simulink model "AFPSM"  (R2018a)
settings: Solver=ode15s  StartTime=0.0  StopTime=5.0  RelTol=1e-3
InitFcn:
  | Pref=2000;
  | D=4;
  | P=10;
  | Rd=5;
  | Rq=5;
  | Ld=2.094;
  | Lq= 0.8187;
  | Phi= 1.6
  | Pref = 2000;
  | J=4;
  | K=0.16;
  | c1= 0.5176;
  | c2= 116;
  | c3= 0.4;
  | c4= 5;
  | c5= 21;
  | c6= 0.0068;
  | Den= 1.225;
  | A= 2
libraries: powerlib x29, simulink x6, powerlib_meascontrol x3
settings Model: Creator=samue  LastModifiedBy=samue

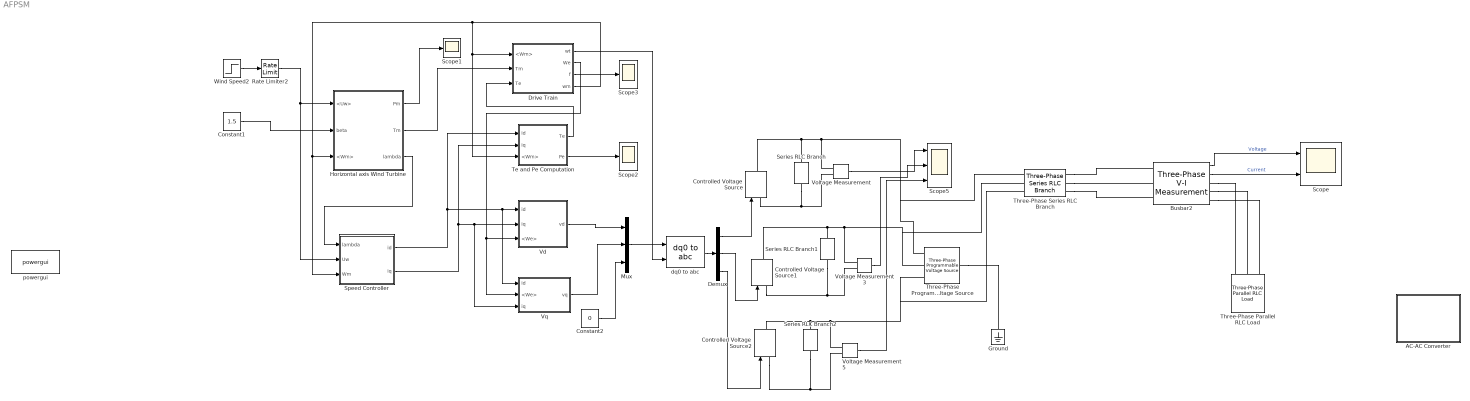
== system AFPSM ==
  AC-AC Converter : Subsystem
  Busbar2 : powerlib/Measurements/Three-Phase V-I Measurement  VoltageMeasurement=phase-to-phase  SetLabelV=off  LabelV=Vabc  Vpu=off  VpuLL=off  CurrentMeasurement=yes  SetLabelI=off  LabelI=Iabc  Ipu=off  Pbase=100e6  Vbase=500e3  OutputType=Complex  PhasorSimulation=off  PSBequivalent=0
  Constant1 : Constant  Value=1.5
  Constant2 : Constant  Value=0
  Controlled Voltage Source : powerlib/Electrical Sources/Controlled Voltage Source  Initialize=on  Source_Type=AC  Amplitude=0  Phase=0  Frequency=60  Measurements=None
  Controlled Voltage Source1 : powerlib/Electrical Sources/Controlled Voltage Source  Initialize=on  Source_Type=AC  Amplitude=0  Phase=0  Frequency=60  Measurements=None
  Controlled Voltage Source2 : powerlib/Electrical Sources/Controlled Voltage Source  Initialize=on  Source_Type=AC  Amplitude=0  Phase=0  Frequency=60  Measurements=None
  Demux : Demux  Outputs=3
  Drive Train : Subsystem
  Ground : powerlib/Elements/Ground  LConnTagsString=a
  Horizontal axis Wind Turbine : Subsystem
  Mux : Mux  Inputs=3
  Rate Limiter2 : RateLimiter
  Scope : Scope  NumInputPorts=2
  Scope1 : Scope
  Scope2 : Scope
  Scope3 : Scope
  Scope5 : Scope  NumInputPorts=3
  Series RLC Branch : powerlib/Elements/Series RLC Branch  LConnTagsString=__new0  RConnTagsString=__new0  BranchType=R  Resistance=1  Inductance=1e-3  SetiL0=off  InitialCurrent=0  Capacitance=1e-6  Setx0=off  InitialVoltage=0  Measurements=None
  Series RLC Branch1 : powerlib/Elements/Series RLC Branch  LConnTagsString=__new0  RConnTagsString=__new0  BranchType=R  Resistance=1  Inductance=1e-3  SetiL0=off  InitialCurrent=0  Capacitance=1e-6  Setx0=off  InitialVoltage=0  Measurements=None
  Series RLC Branch2 : powerlib/Elements/Series RLC Branch  LConnTagsString=__new0  RConnTagsString=__new0  BranchType=R  Resistance=1  Inductance=1e-3  SetiL0=off  InitialCurrent=0  Capacitance=1e-6  Setx0=off  InitialVoltage=0  Measurements=None
  Speed Controller : Subsystem
  Te and Pe Computation : Subsystem
  Three-Phase Parallel RLC Load : powerlib/Elements/Three-Phase Parallel RLC Load  LConnTagsString=A|B|C  Configuration=Y (grounded)  NominalVoltage=1000  Vabc=[1e3 1e3 1e3]  Vabcp=[1e3 1e3 1e3]  NominalFrequency=60  UnbalancedPower=off  ActivePower=10e3  InductivePower=0  CapacitivePower=0  Pabc=[10e3 9e3 11e3]  QLabc=[100 90 110]  QCabc=[100 90 110]  Pabcp=[10e3 9e3 11e3]  QLabcp=[100 90 110]  QCabcp=[100 90 110]  Measurements=None  LoadType=constant Z
  Three-Phase Programmable Voltage Source : powerlib/Electrical Sources/Three-Phase Programmable Voltage Source  PositiveSequence="[100  0 60]"  VariationEntity=None  VariationType=Table of time-amplitude pairs  VariationTypeAlt=Step  VariationStep=0.5  VariationRate=10  VariationMagnitude=0.3  VariationFrequency=2  VariationTiming=[1 2]  VariationPhaseA=off  Amplitudes=[1 0.8 1.2 1.0]  TimeValues=[0 0.1 0.15 0.2]  HarmonicGeneration=off  HarmonicA=[3 0.2 -25 0]  HarmonicB=[2 0.15 35 2]  Timing="[0.05  3]"  BusType=swing  Pref=0  Qref=0  Qmin=-inf  Qmax=inf
  Three-Phase Series RLC Branch : powerlib/Elements/Three-Phase Series RLC Branch  LConnTagsString=A|B|C  RConnTagsString=A|B|C  BranchType=RL  Resistance=1  Inductance=1e-3  Capacitance=1e-6  Measurements=None
  Vd : Subsystem
  Voltage Measurement : powerlib/Measurements/Voltage Measurement  PhasorSimulation=off  OutputType=Complex  PSBequivalent=0
  Voltage Measurement3 : powerlib/Measurements/Voltage Measurement  PhasorSimulation=off  OutputType=Complex  PSBequivalent=0
  Voltage Measurement5 : powerlib/Measurements/Voltage Measurement  PhasorSimulation=off  OutputType=Complex  PSBequivalent=0
  Vq : Subsystem
  Wind Speed2 : Step  Time=2  Before=6  After=15  SampleTime=0
  dq0 to abc : powerlib_meascontrol/Transformations/dq0 to abc  Alignment=90 degrees behind phase A axis
  powergui : powerlib/powergui  Priority=1  SimulationMode=Discrete  SampleTime=50e-6  frequency=60  Iterations=50  frequencyindice=60  Pbase=100e6  ErrMax=1e-4  UnitsV=kV  UnitsW=MW  buscounter=0  FunctionMessages=off  echomessages=off  EnableUseOfTLC=off  CurrentSourceSwitches=off  DisableSnubberDevices=off  DisableRonSwitches=off  DisableVfSwitches=off  DisplayEquations=off  SolverType=Tustin/Backward Euler (TBE)  Interpol=off  ExternalGateDelay=off  methode=off  Ts=100  x0status=blocks  SPID=on  SwTol=0  HookPort=off  RestoreLinks=warning  ResistiveCurrentMeasurement=off  Frange=[0:2:500]  Ylog=off  Xlog=on  ShowGrid=off  save=off  variable=ZData  structure=0  ZoomFFT=off  StartTime=0.0  cycles=1  DisplayStyle=1  fundamental=60  FreqAxis=off  MaxFrequency=1000  frequencyindicesteady=1  RmsSteady=1  display=off
  wires:
  Wind Speed2/1 -> Rate Limiter2/1
  Rate Limiter2/1 -> Speed Controller/2(Uw), Horizontal axis Wind Turbine/1(<Uw>)
  Horizontal axis Wind Turbine/3(lambda) -> Speed Controller/1(lambda)
  Horizontal axis Wind Turbine/2(Tm) -> Drive Train/2(Tm)
  Drive Train/2(We) -> Vd/3(<We>), Vq/2(<We>)
  Speed Controller/1(id) -> Vq/1(id), Vd/1(id), Te and Pe Computation/1(id)
  Speed Controller/2(iq) -> Vq/3(iq), Vd/2(iq), Te and Pe Computation/2(iq)
  Drive Train/4(wm) -> Speed Controller/3(Wm), Horizontal axis Wind Turbine/3(<Wm>), Drive Train/1(<Wm>), Te and Pe Computation/3(<Wm>)
  Te and Pe Computation/1(Te) -> Drive Train/3(Te)
  Constant1/1 -> Horizontal axis Wind Turbine/2(beta)
  Vd/1(vd) -> Mux/1
  Vq/1(vq) -> Mux/2
  Constant2/1 -> Mux/3
  Horizontal axis Wind Turbine/1(Pm) -> Scope1/1
  Drive Train/3(f) -> Scope3/1
  Mux/1 -> dq0 to abc/1
  Drive Train/1(wt) -> dq0 to abc/2
  Te and Pe Computation/2(Pe) -> Scope2/1
  dq0 to abc/1 -> Demux/1
  Demux/1 -> Controlled Voltage Source/1
  Demux/3 -> Controlled Voltage Source2/1
  Demux/2 -> Controlled Voltage Source1/1
  Voltage Measurement/1 -> Scope5/1
  Voltage Measurement3/1 -> Scope5/2
  Voltage Measurement5/1 -> Scope5/3
  Busbar2/2 -> Scope/2  "Current"
  Busbar2/1 -> Scope/1  "Voltage"
  connections:
  Three-Phase Programmable Voltage Source/LConn1 -- Ground/LConn1
  Voltage Measurement/LConn1 -- Three-Phase Series RLC Branch/LConn1 -- Three-Phase Programmable Voltage Source/RConn1 -- Controlled Voltage Source/RConn1 -- Series RLC Branch/LConn1
  Series RLC Branch/RConn1 -- Controlled Voltage Source/LConn1 -- Voltage Measurement/LConn2
  Voltage Measurement3/LConn1 -- Three-Phase Series RLC Branch/LConn2 -- Three-Phase Programmable Voltage Source/RConn2 -- Controlled Voltage Source1/RConn1 -- Series RLC Branch1/LConn1
  Controlled Voltage Source1/LConn1 -- Series RLC Branch1/RConn1 -- Voltage Measurement3/LConn2
  Voltage Measurement5/LConn1 -- Three-Phase Series RLC Branch/LConn3 -- Three-Phase Programmable Voltage Source/RConn3 -- Controlled Voltage Source2/RConn1 -- Series RLC Branch2/LConn1
  Controlled Voltage Source2/LConn1 -- Series RLC Branch2/RConn1 -- Voltage Measurement5/LConn2
  Busbar2/RConn3 -- Three-Phase Parallel RLC Load/LConn3
  Busbar2/RConn2 -- Three-Phase Parallel RLC Load/LConn2
  Busbar2/RConn1 -- Three-Phase Parallel RLC Load/LConn1
  Three-Phase Series RLC Branch/RConn1 -- Busbar2/LConn1
  Three-Phase Series RLC Branch/RConn2 -- Busbar2/LConn2
  Three-Phase Series RLC Branch/RConn3 -- Busbar2/LConn3

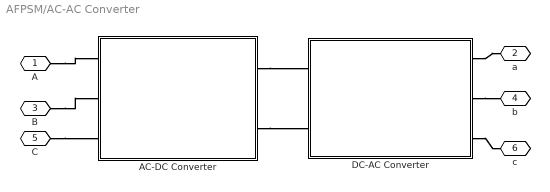
== system AFPSM/AC-AC Converter ==
  AC-DC Converter : Subsystem
  DC-AC Converter : Subsystem
  A : PMIOPort  Side=Left
  a : PMIOPort  Port=2  Side=Right
  B : PMIOPort  Port=3  Side=Left
  b : PMIOPort  Port=4  Side=Right
  C : PMIOPort  Port=5  Side=Left
  c : PMIOPort  Port=6  Side=Right
  connections:
  DC-AC Converter/RConn3 -- c/RConn1
  DC-AC Converter/RConn2 -- b/RConn1
  DC-AC Converter/RConn1 -- a/RConn1
  A/RConn1 -- AC-DC Converter/LConn1
  B/RConn1 -- AC-DC Converter/LConn2
  C/RConn1 -- AC-DC Converter/LConn3
  AC-DC Converter/RConn1 -- DC-AC Converter/LConn1
  AC-DC Converter/RConn2 -- DC-AC Converter/LConn2

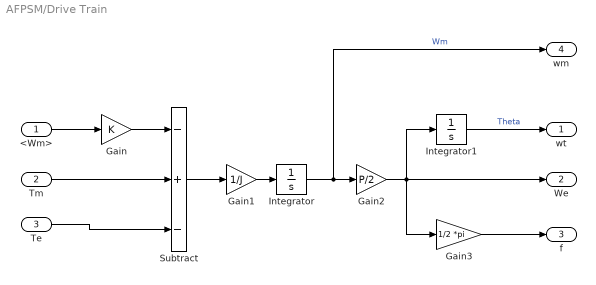
== system AFPSM/Drive Train ==
  <Wm> : Inport
  Tm : Inport  Port=2
  Te : Inport  Port=3
  Gain : Gain  Gain=K
  Gain1 : Gain  Gain=1/J
  Gain2 : Gain  Gain=P/2
  Gain3 : Gain  Gain=1/2 *pi
  Integrator : Integrator
  Integrator1 : Integrator
  Subtract : Sum  Inputs=-+-
  wt : Outport
  We : Outport  Port=2
  f : Outport  Port=3
  wm : Outport  Port=4
  wires:
  Tm/1 -> Subtract/2
  Integrator/1 -> wm/1, Gain2/1  "Wm"
  Gain/1 -> Subtract/1
  Gain2/1 -> We/1, Integrator1/1, Gain3/1
  Te/1 -> Subtract/3
  <Wm>/1 -> Gain/1
  Gain1/1 -> Integrator/1
  Subtract/1 -> Gain1/1
  Integrator1/1 -> wt/1  "Theta"
  Gain3/1 -> f/1

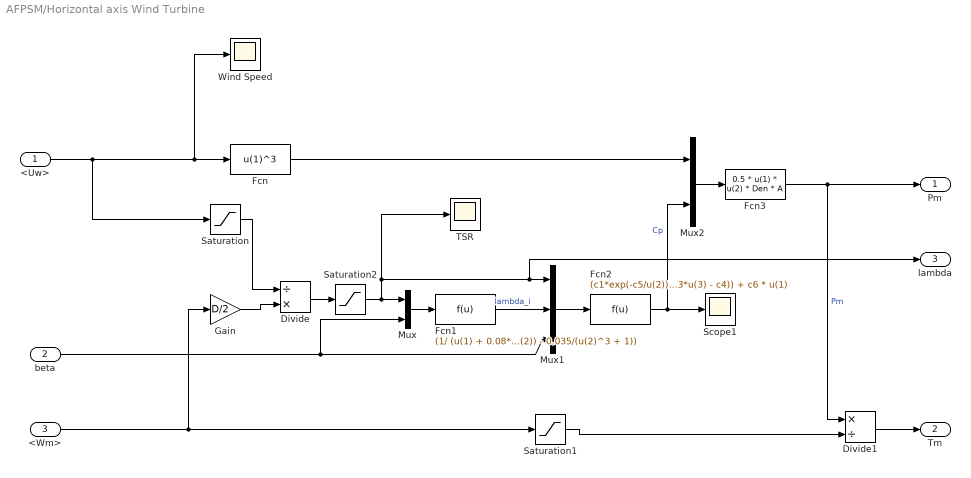
== system AFPSM/Horizontal axis Wind Turbine ==
  <Uw> : Inport
  beta : Inport  Port=2
  <Wm> : Inport  Port=3
  Divide : Product  Inputs=/*
  Divide1 : Product  Inputs=*/
  Fcn : Fcn  Expr=u(1)^3
  Fcn1 : Fcn  Expr=(1/ (u(1) + 0.08*u(2)) - 0.035/(u(2)^3 + 1))
  Fcn2 : Fcn  Expr=(c1*exp(-c5/u(2))*(c2/u(2) - c3*u(3) - c4)) + c6 * u(1)
  Fcn3 : Fcn  Expr=0.5 * u(1) * u(2) * Den * A
  Gain : Gain  Gain=D/2
  Mux : Mux  Inputs=2
  Mux1 : Mux  Inputs=3
  Mux2 : Mux  Inputs=2
  Saturation : Saturate
  Saturation1 : Saturate  UpperLimit=1e6  LowerLimit=1e-6
  Saturation2 : Saturate  UpperLimit=inf  LowerLimit=1e-6
  Scope1 : Scope
  TSR : Scope
  Wind Speed : Scope
  Pm : Outport
  Tm : Outport  Port=2
  lambda : Outport  Port=3
  wires:
  beta/1 -> Mux/2, Mux1/3
  Fcn2/1 -> Scope1/1, Mux2/2  "Cp"
  Divide/1 -> Saturation2/1
  Saturation2/1 -> Mux/1, lambda/1, Mux1/1, TSR/1
  Gain/1 -> Divide/2
  Fcn3/1 -> Pm/1, Divide1/1  "Pm"
  <Uw>/1 -> Saturation/1, Wind Speed/1, Fcn/1
  Mux/1 -> Fcn1/1
  Saturation1/1 -> Divide1/2
  Fcn1/1 -> Mux1/2  "lambda_i"
  <Wm>/1 -> Saturation1/1, Gain/1
  Mux1/1 -> Fcn2/1
  Mux2/1 -> Fcn3/1
  Fcn/1 -> Mux2/1
  Divide1/1 -> Tm/1
  Saturation/1 -> Divide/1

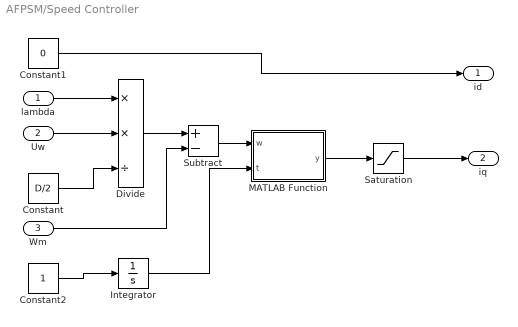
== system AFPSM/Speed Controller ==
  lambda : Inport
  Uw : Inport  Port=2
  Wm : Inport  Port=3
  Constant : Constant  Value=D/2
  Constant1 : Constant  Value=0
  Constant2 : Constant
  Divide : Product  Inputs=**/
  Integrator : Integrator
  MATLAB Function : MATLAB Function  TreatAsAtomicUnit=on
  Saturation : Saturate
  Subtract : Sum  Inputs=+-
  id : Outport
  iq : Outport  Port=2
  wires:
  MATLAB Function/1(y) -> Saturation/1
  Divide/1 -> Subtract/1
  Integrator/1 -> MATLAB Function/2(t)
  Saturation/1 -> iq/1
  Constant2/1 -> Integrator/1
  Constant/1 -> Divide/3
  Wm/1 -> Subtract/2
  Uw/1 -> Divide/2
  Constant1/1 -> id/1
  Subtract/1 -> MATLAB Function/1(w)
  lambda/1 -> Divide/1

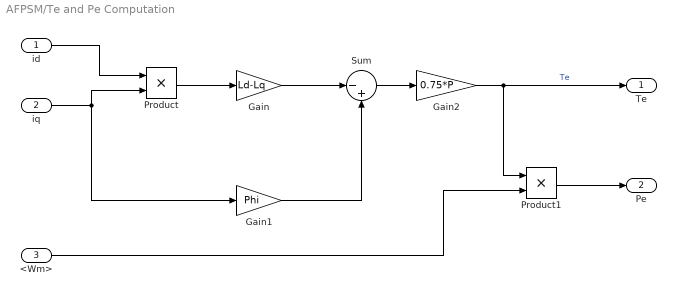
== system AFPSM/Te and Pe Computation ==
  id : Inport
  iq : Inport  Port=2
  <Wm> : Inport  Port=3
  Gain : Gain  Gain=Ld-Lq
  Gain1 : Gain  Gain=Phi
  Gain2 : Gain  Gain=0.75*P
  Product : Product
  Product1 : Product
  Sum : Sum  Inputs=|-+
  Te : Outport
  Pe : Outport  Port=2
  wires:
  <Wm>/1 -> Product1/2
  Product/1 -> Gain/1
  Sum/1 -> Gain2/1
  Gain/1 -> Sum/1
  Gain2/1 -> Te/1, Product1/1  "Te"
  Gain1/1 -> Sum/2
  Product1/1 -> Pe/1
  iq/1 -> Gain1/1, Product/2
  id/1 -> Product/1

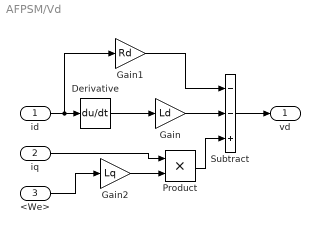
== system AFPSM/Vd ==
  id : Inport
  iq : Inport  Port=2
  <We> : Inport  Port=3
  Derivative : Derivative
  Gain : Gain  Gain=Ld
  Gain1 : Gain  Gain=Rd
  Gain2 : Gain  Gain=Lq
  Product : Product
  Subtract : Sum  Inputs=--+
  vd : Outport
  wires:
  Derivative/1 -> Gain/1
  Gain1/1 -> Subtract/1
  iq/1 -> Product/1
  Subtract/1 -> vd/1
  id/1 -> Gain1/1, Derivative/1
  Product/1 -> Subtract/3
  <We>/1 -> Gain2/1
  Gain/1 -> Subtract/2
  Gain2/1 -> Product/2

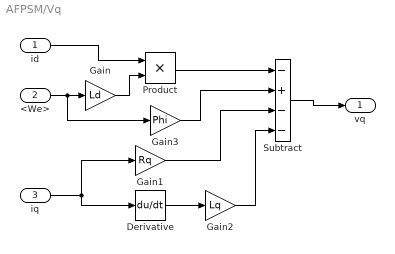
== system AFPSM/Vq ==
  id : Inport
  <We> : Inport  Port=2
  iq : Inport  Port=3
  Derivative : Derivative
  Gain : Gain  Gain=Ld
  Gain1 : Gain  Gain=Rq
  Gain2 : Gain  Gain=Lq
  Gain3 : Gain  Gain=Phi
  Product : Product
  Subtract : Sum  Inputs=-+--
  vq : Outport
  wires:
  iq/1 -> Gain1/1, Derivative/1
  Product/1 -> Subtract/1
  Gain/1 -> Product/2
  Subtract/1 -> vq/1
  <We>/1 -> Gain3/1, Gain/1
  id/1 -> Product/1
  Gain3/1 -> Subtract/2
  Gain1/1 -> Subtract/3
  Gain2/1 -> Subtract/4
  Derivative/1 -> Gain2/1

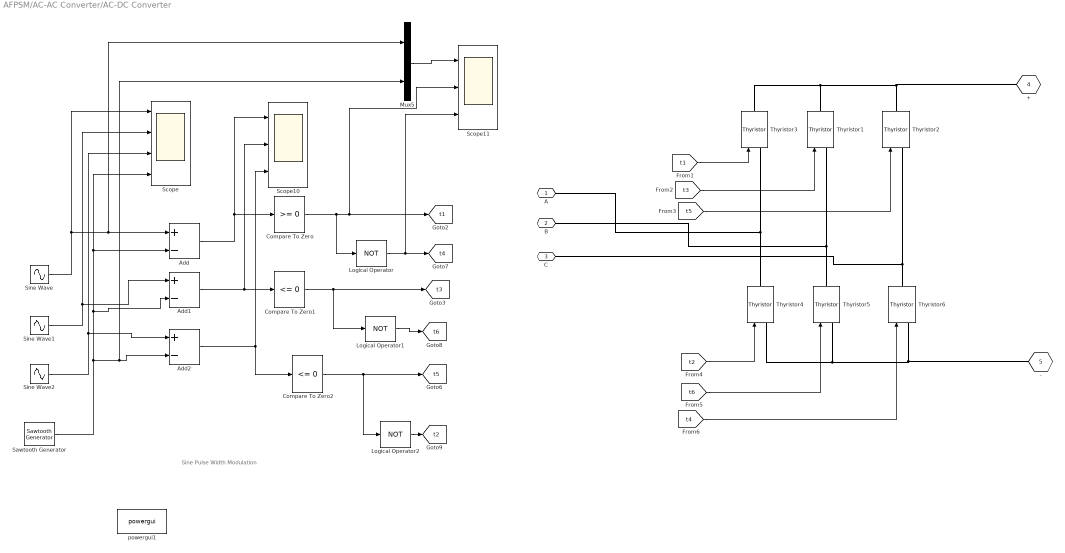
== system AFPSM/AC-AC Converter/AC-DC Converter ==
  note: Sine Pulse Width Modulation
  Add : Sum  Inputs=+-
  Add1 : Sum  Inputs=+-
  Add2 : Sum  Inputs=+-
  Compare To Zero : simulink/Logic and Bit Operations/Compare To Zero  relop=>=  OutDataTypeStr=boolean
  Compare To Zero1 : simulink/Logic and Bit Operations/Compare To Zero  relop=<=  OutDataTypeStr=boolean
  Compare To Zero2 : simulink/Logic and Bit Operations/Compare To Zero  relop=<=  OutDataTypeStr=boolean
  Logical Operator : Logic  Operator=NOT  AllPortsSameDT=off  OutDataTypeStr=boolean
  Logical Operator1 : Logic  Operator=NOT  AllPortsSameDT=off  OutDataTypeStr=boolean
  Logical Operator2 : Logic  Operator=NOT  AllPortsSameDT=off  OutDataTypeStr=boolean
  Mux5 : Mux  Inputs=2
  Sawtooth Generator : powerlib_meascontrol/Pulse & Signal Generators/Sawtooth Generator  Freq=10  Phase=180  Ts=0
      settings: SourceProductName=Simscape Power Systems
  Scope : Scope  NumInputPorts=4
  Scope10 : Scope  NumInputPorts=3
  Scope11 : Scope  NumInputPorts=3
  Sine Wave : Sin  Frequency=2*pi*60  SampleTime=0
  Sine Wave1 : Sin  Frequency=2*pi*60  Phase=(2*pi)/3  SampleTime=0
  Sine Wave2 : Sin  Frequency=2*pi*60  Phase=(-2*pi)/3  SampleTime=0
  Thyristor{1..6} (6 alike) : powerlib/Power Electronics/Thyristor  Ron=0.001  Lon=0  Vf=0.8  IC=0  Rs=500  Cs=250e-9  Measurements=off
  powergui1 : powerlib/powergui  Priority=1  SimulationMode=Continuous  SampleTime=50e-6  frequency=60  Iterations=50  frequencyindice=0  Pbase=100e6  ErrMax=1e-4  UnitsV=kV  UnitsW=MW  buscounter=0  FunctionMessages=off  echomessages=off  EnableUseOfTLC=off  CurrentSourceSwitches=off  DisableSnubberDevices=off  DisableRonSwitches=off  DisableVfSwitches=off  DisplayEquations=off  SolverType=Tustin/Backward Euler (TBE)  Interpol=off  ExternalGateDelay=off  methode=off  Ts=100  x0status=blocks  SPID=on  SwTol=0  HookPort=off  RestoreLinks=warning  ResistiveCurrentMeasurement=off  Frange=[0:2:500]  Ylog=off  Xlog=on  ShowGrid=off  save=off  variable=ZData  structure=0  ZoomFFT=off  StartTime=0.0  cycles=1  DisplayStyle=1  fundamental=60  FreqAxis=off  MaxFrequency=1000  frequencyindicesteady=1  RmsSteady=1  display=off
  A : PMIOPort  Side=Left
  B : PMIOPort  Port=2  Side=Left
  C : PMIOPort  Port=3  Side=Left
  + : PMIOPort  Port=4  Side=Right
  - : PMIOPort  Port=5  Side=Right
  tag scope: t1=global, t2=global, t3=global, t4=global, t5=global, t6=global
  wires:
  [t5] -> Thyristor2/1
  Logical Operator/1 -> Scope11/3, [t4]
  [t2] -> Thyristor4/1
  Sawtooth Generator/1 -> Mux5/2, Add2/2, Add1/2, Add/2, Scope/4
  Sine Wave1/1 -> Add1/1, Scope/2
  Compare To Zero/1 -> [t1], Scope11/2, Logical Operator/1
  Mux5/1 -> Scope11/1
  [t4] -> Thyristor6/1
  Logical Operator1/1 -> [t6]
  Sine Wave/1 -> Mux5/1, Add/1, Scope/1
  Add2/1 -> Compare To Zero2/1, Scope10/3
  Logical Operator2/1 -> [t2]
  Add1/1 -> Compare To Zero1/1, Scope10/2
  Add/1 -> Scope10/1, Compare To Zero/1
  Compare To Zero1/1 -> Logical Operator1/1, [t3]
  [t1] -> Thyristor3/1
  Sine Wave2/1 -> Add2/1, Scope/3
  Compare To Zero2/1 -> Logical Operator2/1, [t5]
  [t3] -> Thyristor1/1
  [t6] -> Thyristor5/1
  connections:
  Thyristor2/RConn1 -- +/RConn1 -- Thyristor1/RConn1 -- Thyristor3/RConn1
  Thyristor4/LConn1 -- Thyristor5/LConn1 -- -/RConn1 -- Thyristor6/LConn1
  Thyristor3/LConn1 -- A/RConn1 -- Thyristor4/RConn1
  Thyristor6/RConn1 -- C/RConn1 -- Thyristor2/LConn1
  Thyristor5/RConn1 -- B/RConn1 -- Thyristor1/LConn1

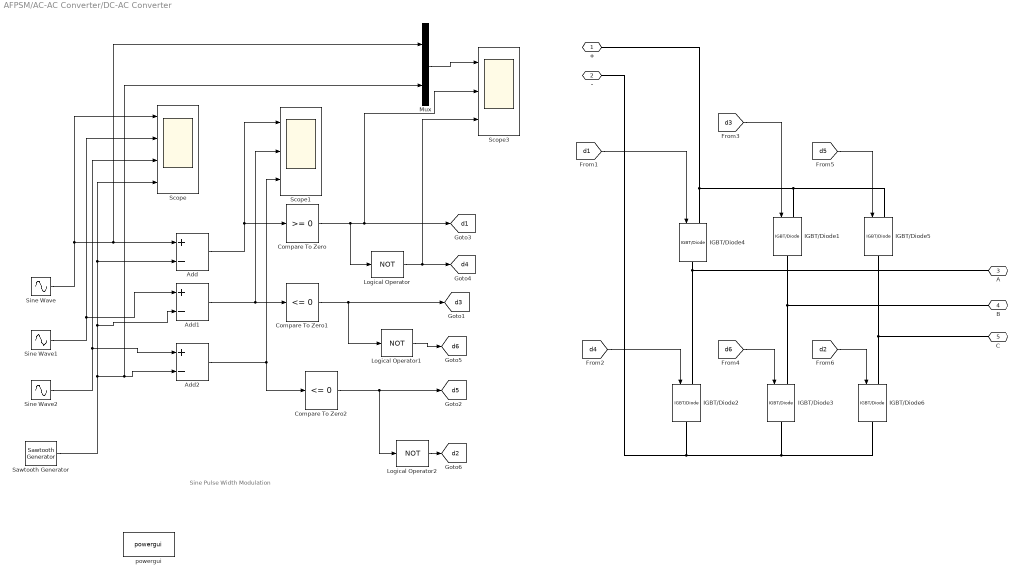
== system AFPSM/AC-AC Converter/DC-AC Converter ==
  note: Sine Pulse Width Modulation
  Add : Sum  Inputs=+-
  Add1 : Sum  Inputs=+-
  Add2 : Sum  Inputs=+-
  Compare To Zero : simulink/Logic and Bit Operations/Compare To Zero  relop=>=  OutDataTypeStr=boolean
  Compare To Zero1 : simulink/Logic and Bit Operations/Compare To Zero  relop=<=  OutDataTypeStr=boolean
  Compare To Zero2 : simulink/Logic and Bit Operations/Compare To Zero  relop=<=  OutDataTypeStr=boolean
  IGBT/Diode{1..6} (6 alike) : powerlib/Power Electronics/IGBT//Diode  Ron=1e-3  Rs=1e5  Cs=inf  Measurements=off
  Logical Operator : Logic  Operator=NOT  AllPortsSameDT=off  OutDataTypeStr=boolean
  Logical Operator1 : Logic  Operator=NOT  AllPortsSameDT=off  OutDataTypeStr=boolean
  Logical Operator2 : Logic  Operator=NOT  AllPortsSameDT=off  OutDataTypeStr=boolean
  Mux : Mux  Inputs=2
  Sawtooth Generator : powerlib_meascontrol/Pulse & Signal Generators/Sawtooth Generator  Freq=10  Phase=180  Ts=0
      settings: SourceProductName=Simscape Power Systems
  Scope : Scope  NumInputPorts=4
  Scope1 : Scope  NumInputPorts=3
  Scope3 : Scope  NumInputPorts=3
  Sine Wave : Sin  Frequency=2*pi*60  SampleTime=0
  Sine Wave1 : Sin  Frequency=2*pi*60  Phase=(2*pi)/3  SampleTime=0
  Sine Wave2 : Sin  Frequency=2*pi*60  Phase=(-2*pi)/3  SampleTime=0
  powergui : powerlib/powergui  Priority=1  SimulationMode=Continuous  SampleTime=50e-6  frequency=60  Iterations=50  frequencyindice=0  Pbase=100e6  ErrMax=1e-4  UnitsV=kV  UnitsW=MW  buscounter=0  FunctionMessages=off  echomessages=off  EnableUseOfTLC=off  CurrentSourceSwitches=off  DisableSnubberDevices=off  DisableRonSwitches=off  DisableVfSwitches=off  DisplayEquations=off  SolverType=Tustin/Backward Euler (TBE)  Interpol=off  ExternalGateDelay=off  methode=off  Ts=100  x0status=blocks  SPID=on  SwTol=0  HookPort=off  RestoreLinks=warning  ResistiveCurrentMeasurement=off  Frange=[0:2:500]  Ylog=off  Xlog=on  ShowGrid=off  save=off  variable=ZData  structure=0  ZoomFFT=off  StartTime=0.0  cycles=1  DisplayStyle=1  fundamental=60  FreqAxis=off  MaxFrequency=1000  frequencyindicesteady=1  RmsSteady=1  display=off
  + : PMIOPort  Side=Left
  - : PMIOPort  Port=2  Side=Left
  A : PMIOPort  Port=3  Side=Right
  B : PMIOPort  Port=4  Side=Right
  C : PMIOPort  Port=5  Side=Right
  tag scope: d1=global, d2=global, d3=global, d4=global, d5=global, d6=global
  wires:
  Sawtooth Generator/1 -> Mux/2, Add2/2, Add1/2, Add/2, Scope/4
  Add/1 -> Scope1/1, Compare To Zero/1
  Add1/1 -> Compare To Zero1/1, Scope1/2
  Compare To Zero/1 -> [d1], Scope3/2, Logical Operator/1
  [d6] -> IGBT/Diode3/1
  Compare To Zero1/1 -> Logical Operator1/1, [d3]
  Sine Wave/1 -> Mux/1, Add/1, Scope/1
  Sine Wave2/1 -> Add2/1, Scope/3
  Mux/1 -> Scope3/1
  Compare To Zero2/1 -> Logical Operator2/1, [d5]
  [d2] -> IGBT/Diode6/1
  [d1] -> IGBT/Diode4/1
  [d3] -> IGBT/Diode1/1
  [d4] -> IGBT/Diode2/1
  [d5] -> IGBT/Diode5/1
  Add2/1 -> Compare To Zero2/1, Scope1/3
  Sine Wave1/1 -> Add1/1, Scope/2
  Logical Operator2/1 -> [d2]
  Logical Operator1/1 -> [d6]
  Logical Operator/1 -> Scope3/3, [d4]
  connections:
  IGBT/Diode6/LConn1 -- C/RConn1 -- IGBT/Diode5/RConn1
  IGBT/Diode4/RConn1 -- IGBT/Diode2/LConn1 -- A/RConn1
  IGBT/Diode4/LConn1 -- +/RConn1 -- IGBT/Diode5/LConn1 -- IGBT/Diode1/LConn1
  IGBT/Diode6/RConn1 -- -/RConn1 -- IGBT/Diode2/RConn1 -- IGBT/Diode3/RConn1
  IGBT/Diode3/LConn1 -- B/RConn1 -- IGBT/Diode1/RConn1

== matlab function AFPSM/Speed Controller/MATLAB Function ==
  data: w input; y output; t input
function y = fcn(w, t)

A=80;
Tc= 300;

y = A * w * (1-exp(-t/Tc));
